simulink model "CICdatapowerfrompropagator_LoLaSat"  (R2022b)
settings: Solver=FixedStepAuto  StartTime=0.0  StopTime=t_sim  FixedStep=TimeStep  RelTol=1e-3
undefined symbols (not defined in the file or in its folder): date, eff_ADC1, eff_GPS, eff_OBC, eff_S, eff_UHF, EN_ADCS1, EN_GPS, EN_heat, EN_OBC, EN_S, EN_Thr, EN_UHF, juliandate, km, MODE, orbit, P_ADC, P_GPS, P_OBC, s
libraries: dspmathops x15, vrlib x8, aerolibutil x8, sharedtransform x7, simulink x4, sharedutil x4, simulink_extras x2, aerolibcelestial x1
settings Model: Creator=colpari  LastModifiedBy=lricc
settings SolverCC: AlgebraicLoopSolver=TrustRegion
settings DebuggingCC: UnconnectedInputMsg=warning  UnconnectedOutputMsg=warning  UnconnectedLineMsg=warning  SFMachineParentedDataDiag=warning
settings ModelReferenceCC: EnableRefExpFcnMdlSchedulingChecks=on
settings RTWCC: DLArmComputeVersion=19.05

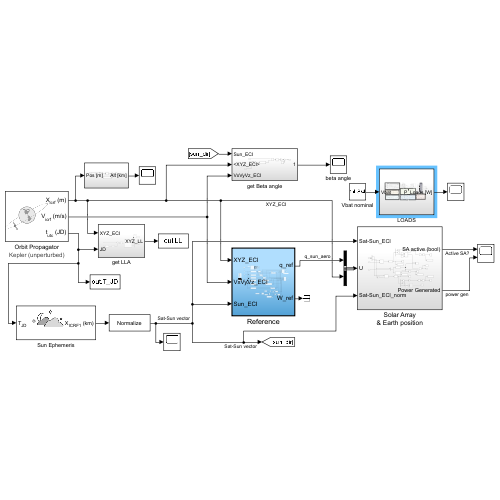
[thumbnail: Simulink's stored preview of the top-level diagram]
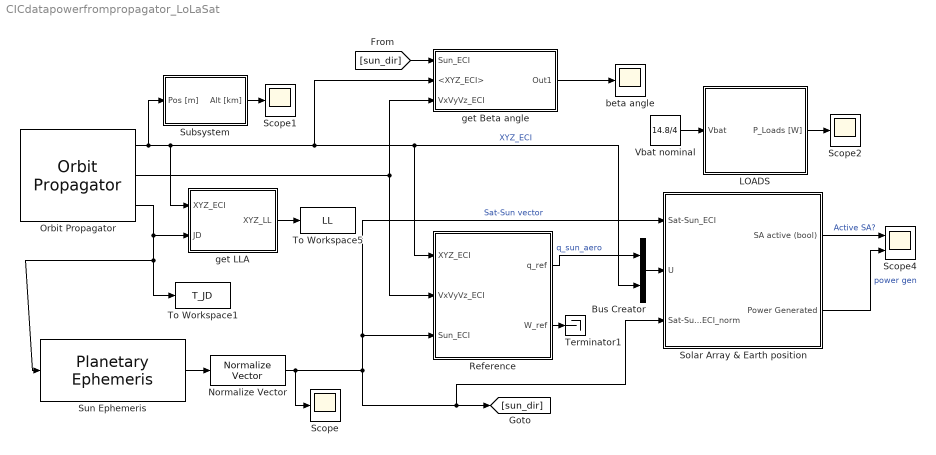
== system CICdatapowerfrompropagator_LoLaSat ==
  Bus Creator : BusCreator  Inputs=2
  LOADS : Subsystem
  Normalize Vector : vrlib/Utilities/Normalize Vector  maxzero=0
  Orbit Propagator : OrbitPropagator  startDate=juliandate(date.year, date.month, date.day, date.hour, date.minutes, date.seconds)  semiMajorAxis=orbit.a  eccentricity=orbit.e  inclination=orbit.i  raan=orbit.O  argPeriapsis=orbit.o  trueAnomaly=orbit.nu  inertialPosition=[3649700.0 3308200.0 -4676600.0]  inertialVelocity=[-2750.8 6666.4 2573.4]  fixedPosition=[-4142689.0 -2676864.7 -4669861.6]  fixedVelocity=[1452.7 -6720.7 2568.1]  customR=3396200  customMu=4.305e13  customJ2=1.0826269e-03  customOmega=4.06125949e-3
      settings: AttributesFormatString=%<propagator>
  Reference : Subsystem  TreatAsAtomicUnit=on
  Scope : Scope
  Scope1 : Scope
  Scope2 : Scope
  Scope4 : Scope  NumInputPorts=2
  Solar Array & Earth position : Subsystem
  Subsystem : Subsystem
  Sun Ephemeris : aerolibcelestial/Planetary Ephemeris  kmflag=km,km/s  epochflag=Julian date  de=DE405  nCenter=Earth  nTarget=Sun  errorflag=Error  velflag=off
  Terminator1 : Terminator
  To Workspace1 : ToWorkspace  VariableName=T_JD  SaveFormat=Timeseries  SampleTime=-1
  To Workspace5 : ToWorkspace  VariableName=LL  SaveFormat=Timeseries  SampleTime=-1
  Vbat nominal : Constant  Value=14.8/4
  beta angle : Scope
  get Beta angle : Subsystem
  get LLA : Subsystem
  wires:
  Reference/1(q_ref) -> Bus Creator/1  "q_sun_aero"
  Solar Array & Earth position/2(Power Generated) -> Scope4/2  "power gen"
  Orbit Propagator/2 -> Reference/2(VxVyVz_ECI), get Beta angle/3(VxVyVz_ECI)
  Normalize Vector/1 -> Scope/1, [sun_dir], Solar Array & Earth position/3(Sat-Sun_ECI_norm), Solar Array & Earth position/1(Sat-Sun_ECI), Reference/3(Sun_ECI)  "Sat-Sun vector"
  Bus Creator/1 -> Solar Array & Earth position/2(U)
  Solar Array & Earth position/1(SA active (bool)) -> Scope4/1  "Active SA?"
  Orbit Propagator/1 -> Subsystem/1(Pos [m]), get LLA/1(XYZ_ECI), Bus Creator/2, Reference/1(XYZ_ECI), get Beta angle/2(<XYZ_ECI>)  "XYZ_ECI"
  Orbit Propagator/3 -> To Workspace1/1, Sun Ephemeris/1, get LLA/2(JD)
  Reference/2(W_ref) -> Terminator1/1
  Sun Ephemeris/1 -> Normalize Vector/1
  get Beta angle/1(Out1) -> beta angle/1
  [sun_dir] -> get Beta angle/1(Sun_ECI)
  Subsystem/1(Alt [km]) -> Scope1/1
  get LLA/1(XYZ_LL) -> To Workspace5/1
  LOADS/1(P_Loads [W]) -> Scope2/1
  Vbat nominal/1 -> LOADS/1(Vbat)

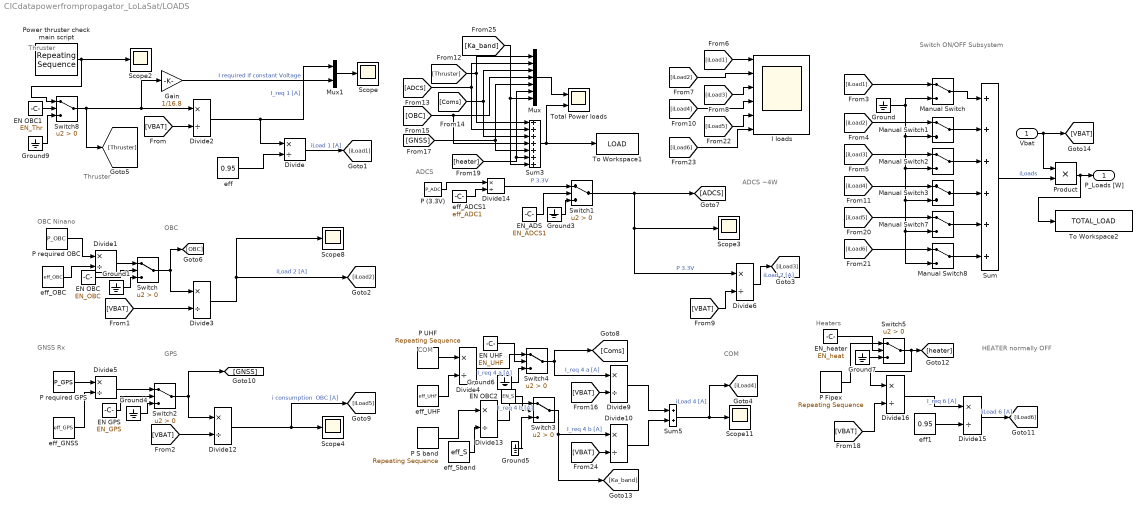
== system CICdatapowerfrompropagator_LoLaSat/LOADS ==
  note: Switch
      | ON/OFF
      | Subsystem
  note: Heaters
  note: COM
  note: ADCS
  note: OBC Ninano
  note: Thruster
  note: ADCS ~4W
  note: COM
  note: Thruster
  note: GNSS Rx
  note: GPS
  note: HEATER
      | normally
      | OFF
  note: OBC
  Vbat : Inport
  Divide{,1..6,9..10,12..16} (14 alike) : Product  Inputs=*/
  EN GPS : Constant  Value=EN_GPS
  EN OBC : Constant  Value=EN_OBC
  EN OBC1 : Constant  Value=EN_Thr
  EN OBC2 : Constant  Value=EN_S
  EN UHF : Constant  Value=EN_UHF
  EN_ADS : Constant  Value=EN_ADCS1
  EN_heater : Constant  Value=EN_heat
  Gain : Gain  Gain=1/16.8
  Ground{,1,3..7,9} (8 alike) : Ground
  I loads : Scope  NumInputPorts=6
  Manual Switch{,1..3,7..8} (6 alike) : ManualSwitch
  Mux : Mux  Inputs=7
  Mux1 : Mux  Inputs=2
  P (3.3V) : Constant  Value=P_ADC
  P Fipex : simulink/Sources/Repeating Sequence  rep_seq_t=t_Fi  rep_seq_y=p_Fi
  "P S band " : simulink/Sources/Repeating Sequence  rep_seq_t=t_tx_S  rep_seq_y=p_tx_S
  "P UHF " : simulink/Sources/Repeating Sequence  rep_seq_t=t_tx_UHF  rep_seq_y=p_tx_UHF
  P required GPS : Constant  Value=P_GPS
  P required OBC : Constant  Value=P_OBC
  Power thruster check main script : simulink/Sources/Repeating Sequence  rep_seq_t=t_thr  rep_seq_y=p_thr
  Product : Product
  Scope{,2..4,8,11} (6 alike) : Scope
  Sum : Sum  Inputs=++++++
  Sum3 : Sum  Inputs=+++++++
  Sum5 : Sum
  Switch{,1..5,8} (7 alike) : Switch  Criteria=u2 > Threshold  SaturateOnIntegerOverflow=off  InputSameDT=off
  To Workspace1 : ToWorkspace  VariableName=LOAD  SaveFormat=Timeseries  SampleTime=-1
  To Workspace2 : ToWorkspace  VariableName=TOTAL_LOAD  SaveFormat=Timeseries  SampleTime=-1
  Total Power loads : Scope  NumInputPorts=2
  eff : Constant  Value=0.95
  eff1 : Constant  Value=0.95
  "eff_ADCS1 " : Constant  Value=eff_ADC1
  eff_GNSS : Constant  Value=eff_GPS
  eff_OBC : Constant  Value=eff_OBC
  eff_Sband : Constant  Value=eff_S
  eff_UHF : Constant  Value=eff_UHF
  P_Loads [W] : Outport
  wires:
  Divide9/1 -> Sum5/1
  Sum5/1 -> [iLoad4], Scope11/1  "iLoad 4 [A]"
  Divide3/1 -> Scope8/1, [iLoad2]  "iLoad 2 [A]"
  Divide14/1 -> Switch1/1  "P 3.3V"
  Ground7/1 -> Switch5/3
  Power thruster check main script/1 -> Scope2/1, Switch8/1
  Sum3/1 -> Total Power loads/2, To Workspace1/1
  [Ka_band] -> Sum3/7, Mux/7
  Mux/1 -> Total Power loads/1
  EN OBC1/1 -> Switch8/2
  Divide4/1 -> Switch4/1  "I_req 4 a [A]"
  Ground5/1 -> Switch3/3
  EN_heater/1 -> Switch5/2
  EN_ADS/1 -> Switch1/2
  Divide10/1 -> Sum5/2
  Ground6/1 -> Switch4/3
  Divide13/1 -> Switch3/1  "I_req 4 b [A]"
  eff_UHF/1 -> Divide4/2
  Divide5/1 -> Switch2/1
  EN UHF/1 -> Switch4/2
  Divide15/1 -> [iLoad6]  "iLoad 6 [A]"
  Divide6/1 -> [iLoad3]  "iLoad 2 [A]"
  EN GPS/1 -> Switch2/2
  EN OBC2/1 -> Switch3/2
  Ground3/1 -> Switch1/3
  [Thruster] -> Sum3/1, Mux/1
  [iLoad6] -> I loads/6
  Manual Switch7/1 -> Sum/5
  Manual Switch8/1 -> Sum/6
  "P UHF "/1 -> Divide4/1
  Divide1/1 -> Switch/1
  eff/1 -> Divide/2
  [VBAT] -> Divide6/2
  Ground4/1 -> Switch2/3
  eff_Sband/1 -> Divide13/2
  [VBAT] -> Divide12/2
  Switch1/1 -> [ADCS], Divide6/1, Scope3/1  "P 3.3V"
  "eff_ADCS1 "/1 -> Divide14/2
  "P S band "/1 -> Divide13/1
  Ground1/1 -> Switch/3
  Switch2/1 -> [GNSS], Divide12/1
  P required OBC/1 -> Divide1/1
  Switch/1 -> Divide3/1, [OBC]
  Switch4/1 -> [Coms], Divide9/1  "I_req 4 a [A]"
  P required GPS/1 -> Divide5/1
  [iLoad3] -> I loads/3
  [iLoad5] -> I loads/5
  [VBAT] -> Divide9/2
  [iLoad6] -> Manual Switch8/1
  P Fipex/1 -> Switch5/1
  Switch8/1 -> [Thruster], Gain/1, Divide2/1
  [GNSS] -> Sum3/5, Mux/5
  [iLoad2] -> I loads/2
  [iLoad5] -> Manual Switch7/1
  Gain/1 -> Mux1/2  "I required if constant Voltage"
  eff_GNSS/1 -> Divide5/2
  [heater] -> Mux/6, Sum3/6
  [VBAT] -> Divide16/2
  Divide16/1 -> Divide15/1  "I_req 6 [A]"
  Divide12/1 -> [iLoad5], Scope4/1  "i consumption  OBC [A]"
  Manual Switch3/1 -> Sum/4
  [iLoad3] -> Manual Switch2/1
  [Coms] -> Sum3/3, Mux/3
  [iLoad4] -> I loads/4
  EN OBC/1 -> Switch/2
  [iLoad2] -> Manual Switch1/1
  [OBC] -> Sum3/4, Mux/4
  eff1/1 -> Divide15/2
  Manual Switch2/1 -> Sum/3
  Switch3/1 -> [Ka_band], Divide10/1  "I_req 4 b [A]"
  Manual Switch/1 -> Sum/1
  [ADCS] -> Sum3/2, Mux/2
  [VBAT] -> Divide10/2
  [iLoad4] -> Manual Switch3/1
  Mux1/1 -> Scope/1
  [iLoad1] -> Manual Switch/1
  Ground/1 -> Manual Switch/2, Manual Switch8/2, Manual Switch7/2, Manual Switch3/2, Manual Switch2/2, Manual Switch1/2
  Switch5/1 -> Divide16/1, [heater]
  Ground9/1 -> Switch8/3
  Divide2/1 -> Divide/1, Mux1/1  "I_req 1 [A]"
  [iLoad1] -> I loads/1
  [VBAT] -> Divide3/2
  Divide/1 -> [iLoad1]  "iLoad 1 [A]"
  eff_OBC/1 -> Divide1/2
  Manual Switch1/1 -> Sum/2
  [VBAT] -> Divide2/2
  P (3.3V)/1 -> Divide14/1
  Product/1 -> To Workspace2/1, P_Loads [W]/1
  Sum/1 -> Product/2  "iLoads"
  Vbat/1 -> Product/1, [VBAT]

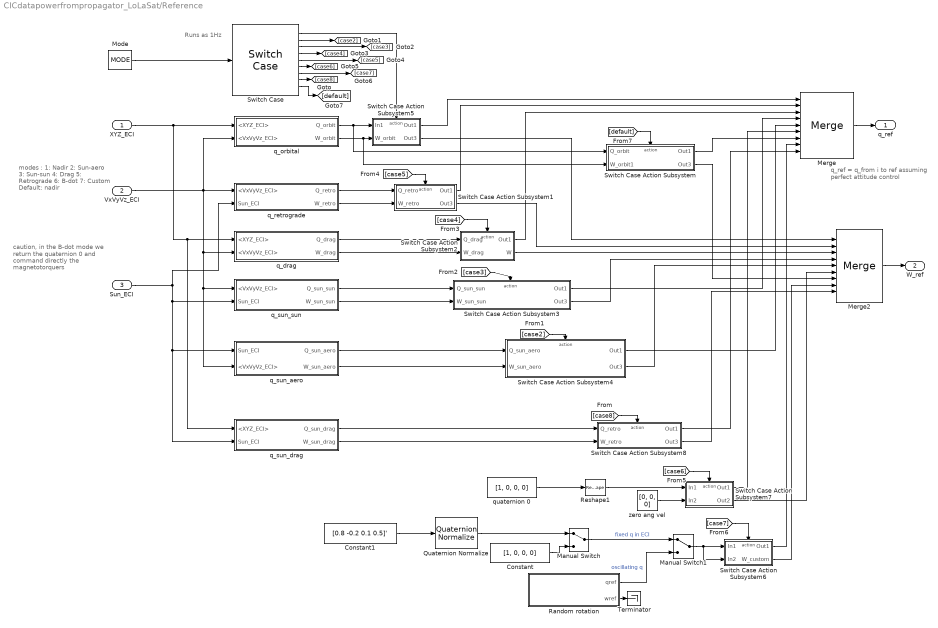
== system CICdatapowerfrompropagator_LoLaSat/Reference ==
  note: caution, in the B-dot mode we return the quaternion 0 and command directly the magnetotorquers
  note: modes :
      | 1: Nadir
      | 2: Sun-aero
      | 3: Sun-sun
      | 4: Drag
      | 5: Retrograde
      | 6: B-dot
      | 7: Custom
      | Default: nadir
  note: Runs as 1Hz
  note: q_ref  = q_from i to ref
      | assuming perfect attitude control
  XYZ_ECI : Inport
  VxVyVz_ECI : Inport  Port=2
  Sun_ECI : Inport  Port=3
  Constant : Constant  Value=[1, 0, 0, 0]
  Constant1 : Constant  Value=[0.8 -0.2 0.1 0.5]'
  Manual Switch : ManualSwitch
  Manual Switch1 : ManualSwitch
  Merge : Merge  Inputs=9
  Merge2 : Merge  Inputs=9
  Mode : Constant  Value=MODE  OutDataTypeStr=int8
  Quaternion Normalize : sharedutil/Quaternion Normalize  aMode=aMode
  Random rotation : Subsystem
  Reshape1 : Reshape  OutputDimensionality=Column vector (2-D)
  Switch Case : SwitchCase  CaseConditions={1, 2, 3, 4, 5, 6, 7, 8}
  Switch Case Action Subsystem : Subsystem  TreatAsAtomicUnit=on
  Switch Case Action Subsystem1 : Subsystem  TreatAsAtomicUnit=on
  Switch Case Action Subsystem2 : Subsystem  TreatAsAtomicUnit=on
  Switch Case Action Subsystem3 : Subsystem  TreatAsAtomicUnit=on
  Switch Case Action Subsystem4 : Subsystem  TreatAsAtomicUnit=on
  Switch Case Action Subsystem5 : Subsystem  TreatAsAtomicUnit=on
  Switch Case Action Subsystem6 : Subsystem  TreatAsAtomicUnit=on
  Switch Case Action Subsystem7 : Subsystem  TreatAsAtomicUnit=on
  Switch Case Action Subsystem8 : Subsystem  TreatAsAtomicUnit=on
  Terminator : Terminator
  q_drag : Subsystem
  q_orbital : Subsystem
  q_retrograde : Subsystem
  q_sun_aero : Subsystem
  q_sun_drag : Subsystem
  q_sun_sun : Subsystem
  quaternion 0 : Constant  Value=[1, 0, 0, 0]
  zero ang vel : Constant  Value=[0, 0, 0]
  q_ref : Outport  VectorParamsAs1DForOutWhenUnconnected=off
  W_ref : Outport  Port=2
  wires:
  q_sun_sun/1(Q_sun_sun) -> Switch Case Action Subsystem3/1(Q_sun_sun)
  Sun_ECI/1 -> q_retrograde/2(Sun_ECI), q_sun_drag/2(Sun_ECI), q_sun_aero/1(Sun_ECI), q_sun_sun/2(Sun_ECI)
  Mode/1 -> Switch Case/1
  q_sun_aero/1(Q_sun_aero) -> Switch Case Action Subsystem4/1(Q_sun_aero)
  Merge/1 -> q_ref/1
  quaternion 0/1 -> Reshape1/1
  VxVyVz_ECI/1 -> q_orbital/2(<VxVyVz_ECI>), q_retrograde/1(<VxVyVz_ECI>), q_drag/2(<VxVyVz_ECI>), q_sun_aero/2(<VxVyVz_ECI>), q_sun_sun/1(<VxVyVz_ECI>)
  q_orbital/1(Q_orbit) -> Switch Case Action Subsystem/1(Q_orbit), Switch Case Action Subsystem5/1(In1)
  q_retrograde/1(Q_retro) -> Switch Case Action Subsystem1/1(Q_retro)
  Reshape1/1 -> Switch Case Action Subsystem7/1(In1)
  Switch Case Action Subsystem5/1(Out1) -> Merge/1
  Switch Case Action Subsystem1/1(Out1) -> Merge/2
  Switch Case Action Subsystem2/1(Out1) -> Merge/3
  Switch Case Action Subsystem3/1(Out1) -> Merge/4
  Switch Case Action Subsystem4/1(Out1) -> Merge/5
  Switch Case Action Subsystem/1(Out1) -> Merge/7
  Switch Case Action Subsystem7/1(Out1) -> Merge/6
  Switch Case/1 -> Switch Case Action Subsystem5/Action
  Constant/1 -> Manual Switch/2
  Switch Case Action Subsystem6/1(Out1) -> Merge/8
  Constant1/1 -> Quaternion Normalize/1
  Quaternion Normalize/1 -> Manual Switch/1
  q_orbital/2(W_orbit) -> Switch Case Action Subsystem/2(W_orbit1), Switch Case Action Subsystem5/2(W_orbit)
  q_retrograde/2(W_retro) -> Switch Case Action Subsystem1/2(W_retro)
  q_sun_aero/2(W_sun_aero) -> Switch Case Action Subsystem4/2(W_sun_aero)
  q_sun_sun/2(W_sun_sun) -> Switch Case Action Subsystem3/2(W_sun_sun)
  Merge2/1 -> W_ref/1
  Switch Case Action Subsystem5/2(Out3) -> Merge2/1
  Switch Case Action Subsystem4/2(Out3) -> Merge2/5
  Switch Case Action Subsystem3/2(Out3) -> Merge2/4
  Switch Case Action Subsystem2/2(W) -> Merge2/3
  Switch Case Action Subsystem1/2(Out3) -> Merge2/2
  zero ang vel/1 -> Switch Case Action Subsystem7/2(In2)
  Switch Case Action Subsystem7/2(Out2) -> Merge2/6
  Switch Case Action Subsystem/2(Out3) -> Merge2/7
  Switch Case Action Subsystem6/2(W_custom) -> Merge2/8
  q_drag/1(Q_drag) -> Switch Case Action Subsystem2/1(Q_drag)
  q_drag/2(W_drag) -> Switch Case Action Subsystem2/2(W_drag)
  Manual Switch/1 -> Manual Switch1/1  "fixed q in ECI"
  Random rotation/1(qref) -> Manual Switch1/2  "oscillating q"
  Manual Switch1/1 -> Switch Case Action Subsystem6/2(In2), Switch Case Action Subsystem6/1(In1)
  Random rotation/2(wref) -> Terminator/1
  XYZ_ECI/1 -> q_sun_drag/1(<XYZ_ECI>), q_drag/1(<XYZ_ECI>), q_orbital/1(<XYZ_ECI>)
  q_sun_drag/1(Q_sun_drag) -> Switch Case Action Subsystem8/1(Q_retro)
  q_sun_drag/2(W_sun_drag) -> Switch Case Action Subsystem8/2(W_retro)
  Switch Case/8 -> [case8]
  [case8] -> Switch Case Action Subsystem8/Action
  Switch Case Action Subsystem8/1(Out1) -> Merge/9
  Switch Case Action Subsystem8/2(Out3) -> Merge2/9
  Switch Case/2 -> [case2]
  [case2] -> Switch Case Action Subsystem4/Action
  Switch Case/3 -> [case3]
  [case3] -> Switch Case Action Subsystem3/Action
  Switch Case/4 -> [case4]
  [case4] -> Switch Case Action Subsystem2/Action
  Switch Case/5 -> [case5]
  [case5] -> Switch Case Action Subsystem1/Action
  Switch Case/6 -> [case6]
  [case6] -> Switch Case Action Subsystem7/Action
  Switch Case/7 -> [case7]
  [case7] -> Switch Case Action Subsystem6/Action
  Switch Case/9 -> [default]
  [default] -> Switch Case Action Subsystem/Action

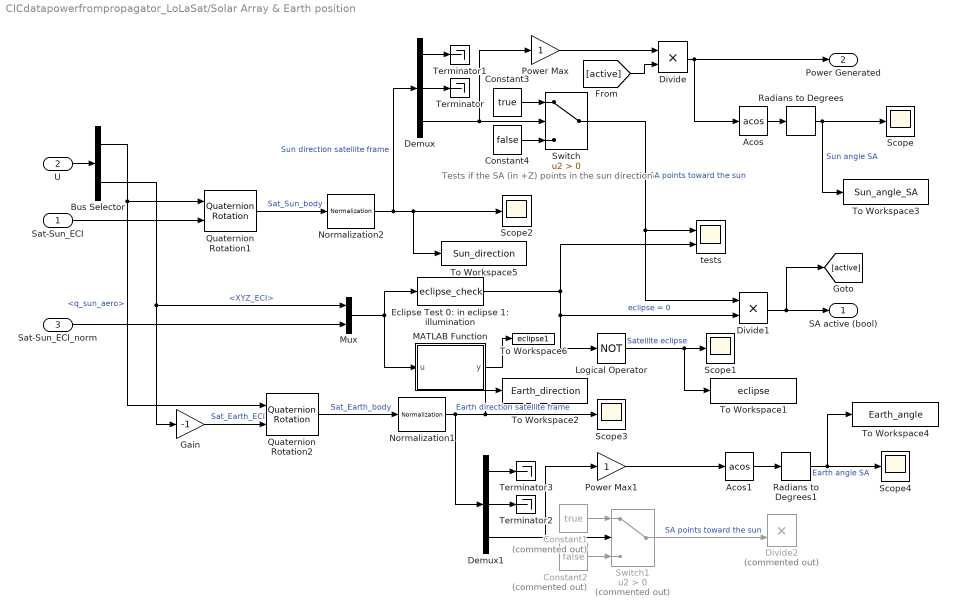
== system CICdatapowerfrompropagator_LoLaSat/Solar Array & Earth position ==
  note: Tests if the SA (in +Z) points in the sun direction
  Sat-Sun_ECI : Inport
  U : Inport  Port=2
  Sat-Sun_ECI_norm : Inport  Port=3
  Acos : Trigonometry  Operator=acos
  Acos1 : Trigonometry  Operator=acos
  Bus Selector : BusSelector  OutputSignals=q_sun_aero,XYZ_ECI
  Constant1 : Constant  Commented=on  Value=true
  Constant2 : Constant  Commented=on  Value=false
  Constant3 : Constant  Value=true
  Constant4 : Constant  Value=false
  Demux : Demux  Outputs=3
  Demux1 : Demux  Outputs=3
  Divide : Product  Inputs=**
  Divide1 : Product  Inputs=**
  Divide2 : Product  Commented=on  Inputs=**
  Eclipse Test 0: in eclipse 1: illumination : MATLABFcn  MATLABFcn=eclipse_check
  Gain : Gain  Gain=-1
  Logical Operator : Logic  Operator=NOT  AllPortsSameDT=off
  MATLAB Function : MATLAB Function  TreatAsAtomicUnit=on
  Mux : Mux  Inputs=2
  Normalization1 : dspmathops/Normalization  NormType=2-norm  Bias=1e-10  NormOver=Each column  Dimension=1  roundingMode=Floor  overflowMode=off  accumDataTypeStr=Inherit: Same as product output  accumLastDataTypeStr=Inherit: Same as product output  outputDataTypeStr=Inherit: Same as product output  outputMin=[]  outputMax=[]  outputLastDataTypeStr=Inherit: Same as product output
  Normalization2 : dspmathops/Normalization  NormType=2-norm  Bias=1e-10  NormOver=Each column  Dimension=1  roundingMode=Floor  overflowMode=off  accumDataTypeStr=Inherit: Same as product output  accumLastDataTypeStr=Inherit: Same as product output  outputDataTypeStr=Inherit: Same as product output  outputMin=[]  outputMax=[]  outputLastDataTypeStr=Inherit: Same as product output
  Power Max : Gain
  Power Max1 : Gain
  Quaternion Rotation1 : aerolibutil/Quaternion Rotation
  Quaternion Rotation2 : aerolibutil/Quaternion Rotation
  Radians to Degrees : simulink_extras/Transformations/Radians to Degrees
  Radians to Degrees1 : simulink_extras/Transformations/Radians to Degrees
  Scope{,1..4} (5 alike) : Scope
  Switch : Switch  Criteria=u2 > Threshold  SaturateOnIntegerOverflow=off  InputSameDT=off
  Switch1 : Switch  Commented=on  Criteria=u2 > Threshold  SaturateOnIntegerOverflow=off  InputSameDT=off
  Terminator{,1..3} (4 alike) : Terminator
  To Workspace1 : ToWorkspace  VariableName=eclipse  SaveFormat=Timeseries  SampleTime=-1
  To Workspace2 : ToWorkspace  VariableName=Earth_direction  SaveFormat=Timeseries  SampleTime=-1
  To Workspace3 : ToWorkspace  VariableName=Sun_angle_SA  SaveFormat=Timeseries  SampleTime=-1
  To Workspace4 : ToWorkspace  VariableName=Earth_angle  SaveFormat=Timeseries  SampleTime=-1
  To Workspace5 : ToWorkspace  VariableName=Sun_direction  SaveFormat=Timeseries  SampleTime=-1
  To Workspace6 : ToWorkspace  VariableName=eclipse1  SaveFormat=Timeseries  SampleTime=-1
  tests : Scope  NumInputPorts=2
  SA active (bool) : Outport  VectorParamsAs1DForOutWhenUnconnected=off
  Power Generated : Outport  Port=2
  wires:
  Switch/1 -> Divide1/1, tests/1  "SA points toward the sun"
  U/1 -> Bus Selector/1
  Sat-Sun_ECI/1 -> Quaternion Rotation1/2
  Bus Selector/1 -> Quaternion Rotation2/1, Quaternion Rotation1/1  "<q_sun_aero>"
  Quaternion Rotation1/1 -> Normalization2/1  "Sat_Sun_body"
  Demux/3 -> Power Max/1, Switch/2
  Constant3/1 -> Switch/1
  Demux/2 -> Terminator/1
  Demux/1 -> Terminator1/1
  Bus Selector/2 -> Gain/1, Mux/1  "<XYZ_ECI>"
  Divide1/1 -> [active], SA active (bool)/1
  Constant4/1 -> Switch/3
  Normalization2/1 -> To Workspace5/1, Scope2/1, Demux/1  "Sun direction satellite frame"
  Divide/1 -> Acos/1, Power Generated/1
  Power Max/1 -> Divide/1
  [active] -> Divide/2
  Sat-Sun_ECI_norm/1 -> Mux/2
  Mux/1 -> Eclipse Test 0: in eclipse 1: illumination/1, MATLAB Function/1(u)
  Eclipse Test 0: in eclipse 1: illumination/1 -> Logical Operator/1, Divide1/2, tests/2  "eclipse = 0"
  Acos/1 -> Radians to Degrees/1
  Radians to Degrees/1 -> To Workspace3/1, Scope/1  "Sun angle SA"
  Logical Operator/1 -> To Workspace1/1, Scope1/1  "Satellite eclipse"
  Gain/1 -> Quaternion Rotation2/2  "Sat_Earth_ECI"
  Quaternion Rotation2/1 -> Normalization1/1  "Sat_Earth_body"
  Power Max1/1 -> Acos1/1
  Demux1/3 -> Power Max1/1, Switch1/2
  Demux1/2 -> Terminator2/1
  Normalization1/1 -> Demux1/1, To Workspace2/1, Scope3/1  "Earth direction satellite frame"
  Constant2/1 -> Switch1/3
  Constant1/1 -> Switch1/1
  Switch1/1 -> Divide2/2  "SA points toward the sun"
  Demux1/1 -> Terminator3/1
  Acos1/1 -> Radians to Degrees1/1
  Radians to Degrees1/1 -> To Workspace4/1, Scope4/1  "Earth angle SA"
  MATLAB Function/1(y) -> To Workspace6/1

== system CICdatapowerfrompropagator_LoLaSat/Subsystem ==
  Pos [m] : Inport
  Constant : Constant  Value=orbit.R_earth
  Dot Product : DotProduct  OutDataTypeStr=Inherit: Inherit via internal rule
  Gain : Gain  Gain=1e-3
  Sqrt : Sqrt
  Sum : Sum  Inputs=|+-
  Alt [km] : Outport
  wires:
  Dot Product/1 -> Sqrt/1
  Pos [m]/1 -> Dot Product/2, Dot Product/1
  Sqrt/1 -> Sum/1
  Constant/1 -> Sum/2
  Sum/1 -> Gain/1
  Gain/1 -> Alt [km]/1

== system CICdatapowerfrompropagator_LoLaSat/get Beta angle ==
  Sun_ECI : Inport
  <XYZ_ECI> : Inport  Port=2
  VxVyVz_ECI : Inport  Port=3
  Acos : Trigonometry  Operator=acos
  Constant1 : Constant  Value=90
  Cross Product : vrlib/Utilities/Cross Product
  Dot Product : DotProduct  OutDataTypeStr=Inherit: Inherit via internal rule
  Gain : Gain  Gain=180/pi
  Normalize Vector2 : vrlib/Utilities/Normalize Vector  maxzero=0
  Sum : Sum  Inputs=|-+
  Out1 : Outport
  wires:
  Normalize Vector2/1 -> Dot Product/2  "x"
  Constant1/1 -> Sum/2
  Cross Product/1 -> Normalize Vector2/1
  Sun_ECI/1 -> Dot Product/1
  Dot Product/1 -> Acos/1
  Acos/1 -> Gain/1
  Gain/1 -> Sum/1
  Sum/1 -> Out1/1
  <XYZ_ECI>/1 -> Cross Product/1
  VxVyVz_ECI/1 -> Cross Product/2

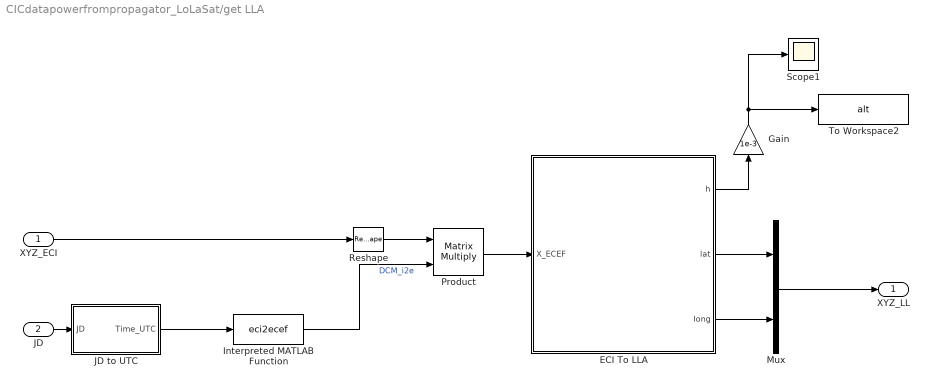
== system CICdatapowerfrompropagator_LoLaSat/get LLA ==
  XYZ_ECI : Inport
  JD : Inport  Port=2
  ECI To LLA : MATLAB Function  TreatAsAtomicUnit=on
  Gain : Gain  Gain=1e-3
  Interpreted MATLAB Function : MATLABFcn  MATLABFcn=eci2ecef  OutputDimensions=[3,3]  Output1D=off
  JD to UTC : MATLAB Function  TreatAsAtomicUnit=on
  Mux : Mux  Inputs=2
  Product : Product  Multiplication=Matrix(*)
  Reshape : Reshape  OutputDimensionality=Row vector (2-D)
  Scope1 : Scope
  To Workspace2 : ToWorkspace  VariableName=alt  SaveFormat=Timeseries  SampleTime=-1
  XYZ_LL : Outport
  wires:
  JD to UTC/1(Time_UTC) -> Interpreted MATLAB Function/1
  JD/1 -> JD to UTC/1(JD)
  Product/1 -> ECI To LLA/1(X_ECEF)
  ECI To LLA/2(lat) -> Mux/1
  ECI To LLA/3(long) -> Mux/2
  ECI To LLA/1(h) -> Gain/1
  Reshape/1 -> Product/1
  XYZ_ECI/1 -> Reshape/1
  Interpreted MATLAB Function/1 -> Product/2  "DCM_i2e"
  Gain/1 -> Scope1/1, To Workspace2/1
  Mux/1 -> XYZ_LL/1

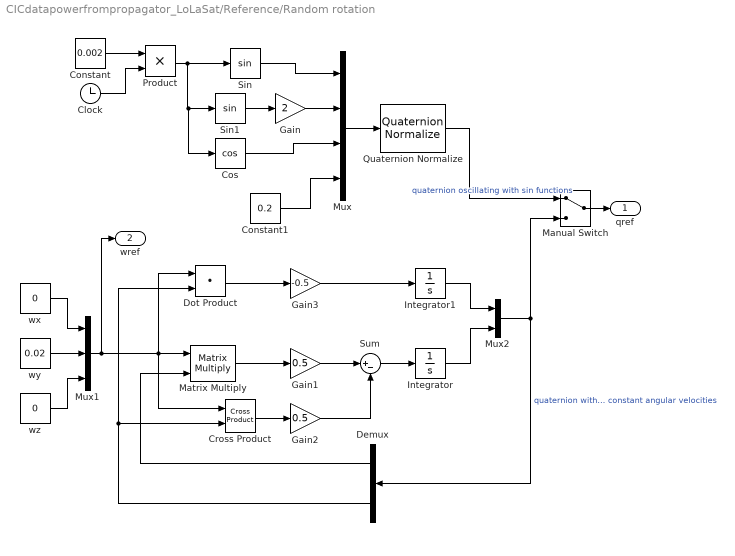
== system CICdatapowerfrompropagator_LoLaSat/Reference/Random rotation ==
  Clock : Clock
      settings: Decimation=TimeStep
  Constant : Constant  Value=0.002
  Constant1 : Constant  Value=0.2
  Cos : Trigonometry  Operator=cos
  Cross Product : vrlib/Utilities/Cross Product
  Demux : Demux  Outputs=[1;3]
  Dot Product : DotProduct  OutDataTypeStr=Inherit: Inherit via internal rule
  Gain : Gain  Gain=2
  Gain1 : Gain  Gain=0.5
  Gain2 : Gain  Gain=0.5
  Gain3 : Gain  Gain=-0.5
  Integrator : Integrator  InitialCondition=[0;0;0]
  Integrator1 : Integrator  InitialCondition=1
  Manual Switch : ManualSwitch
  Matrix Multiply : Product  Multiplication=Matrix(*)
  Mux : Mux
  Mux1 : Mux  Inputs=3
  Mux2 : Mux  Inputs=[1;3]
  Product : Product
  Quaternion Normalize : sharedutil/Quaternion Normalize  aMode=aMode
  Sin : Trigonometry
  Sin1 : Trigonometry
  Sum : Sum  Inputs=|+-
  wx : Constant  Value=0
  wy : Constant  Value=0.02
  wz : Constant  Value=0
  qref : Outport
  wref : Outport  Port=2
  wires:
  Mux/1 -> Quaternion Normalize/1
  Quaternion Normalize/1 -> Manual Switch/1  "quaternion oscillating with sin functions"
  Constant/1 -> Product/1
  Clock/1 -> Product/2
  Product/1 -> Cos/1, Sin1/1, Sin/1
  Sin/1 -> Mux/1
  Sin1/1 -> Gain/1
  Gain/1 -> Mux/2
  Cos/1 -> Mux/3
  Constant1/1 -> Mux/4
  Manual Switch/1 -> qref/1
  wx/1 -> Mux1/1
  wy/1 -> Mux1/2
  wz/1 -> Mux1/3
  Mux1/1 -> wref/1, Dot Product/1, Cross Product/1, Matrix Multiply/1
  Matrix Multiply/1 -> Gain1/1
  Gain1/1 -> Sum/1
  Sum/1 -> Integrator/1
  Integrator/1 -> Mux2/2
  Mux2/1 -> Demux/1, Manual Switch/2  "quaternion with constant angular velocities"
  Demux/1 -> Matrix Multiply/2
  Cross Product/1 -> Gain2/1
  Gain2/1 -> Sum/2
  Dot Product/1 -> Gain3/1
  Gain3/1 -> Integrator1/1
  Integrator1/1 -> Mux2/1
  Demux/2 -> Cross Product/2, Dot Product/2

== system CICdatapowerfrompropagator_LoLaSat/Reference/Switch Case Action Subsystem ==
  Q_orbit : Inport
  W_orbit1 : Inport  Port=2
  Action Port : ActionPort  ActionPortLabel=default:
  Out1 : Outport  VectorParamsAs1DForOutWhenUnconnected=off
  Out3 : Outport  Port=2  VectorParamsAs1DForOutWhenUnconnected=off
  wires:
  Q_orbit/1 -> Out1/1
  W_orbit1/1 -> Out3/1

== system CICdatapowerfrompropagator_LoLaSat/Reference/Switch Case Action Subsystem1 ==
  Q_retro : Inport
  W_retro : Inport  Port=2
  Action Port : ActionPort  ActionPortLabel=case [ 5 ]:
  Out1 : Outport  VectorParamsAs1DForOutWhenUnconnected=off
  Out3 : Outport  Port=2  VectorParamsAs1DForOutWhenUnconnected=off
  wires:
  Q_retro/1 -> Out1/1
  W_retro/1 -> Out3/1

== system CICdatapowerfrompropagator_LoLaSat/Reference/Switch Case Action Subsystem2 ==
  note: q from I to O + rotation
  Q_drag : Inport
  W_drag : Inport  Port=2
  Action Port : ActionPort  ActionPortLabel=case [ 4 ]:
  Out1 : Outport  VectorParamsAs1DForOutWhenUnconnected=off
  W : Outport  Port=2
  wires:
  Q_drag/1 -> Out1/1
  W_drag/1 -> W/1

== system CICdatapowerfrompropagator_LoLaSat/Reference/Switch Case Action Subsystem3 ==
  Q_sun_sun : Inport
  W_sun_sun : Inport  Port=2
  Action Port : ActionPort  ActionPortLabel=case [ 3 ]:
  Out1 : Outport  VectorParamsAs1DForOutWhenUnconnected=off
  Out3 : Outport  Port=2  VectorParamsAs1DForOutWhenUnconnected=off
  wires:
  Q_sun_sun/1 -> Out1/1
  W_sun_sun/1 -> Out3/1

== system CICdatapowerfrompropagator_LoLaSat/Reference/Switch Case Action Subsystem4 ==
  Q_sun_aero : Inport
  W_sun_aero : Inport  Port=2
  Action Port : ActionPort  ActionPortLabel=case [ 2 ]:
  Out1 : Outport  VectorParamsAs1DForOutWhenUnconnected=off
  Out3 : Outport  Port=2  VectorParamsAs1DForOutWhenUnconnected=off
  wires:
  Q_sun_aero/1 -> Out1/1
  W_sun_aero/1 -> Out3/1

== system CICdatapowerfrompropagator_LoLaSat/Reference/Switch Case Action Subsystem5 ==
  In1 : Inport
  W_orbit : Inport  Port=2
  Action Port : ActionPort  ActionPortLabel=case [ 1 ]:
  Out1 : Outport  VectorParamsAs1DForOutWhenUnconnected=off
  Out3 : Outport  Port=2  VectorParamsAs1DForOutWhenUnconnected=off
  wires:
  In1/1 -> Out1/1
  W_orbit/1 -> Out3/1

== system CICdatapowerfrompropagator_LoLaSat/Reference/Switch Case Action Subsystem6 ==
  In1 : Inport
  In2 : Inport  Port=2
  Action Port : ActionPort  ActionPortLabel=case [ 7 ]:
  Derivative : Derivative
  Matrix Multiply : Product  Multiplication=Matrix(*)
  Quaternions to Direction Cosine Matrix : sharedtransform/Quaternions to  Direction Cosine Matrix  aMode=aMode
  Transpose : Math  Operator=transpose
  Transpose1 : Math  Operator=transpose
  gets vector from Skew Matrix : MATLABFcn  MATLABFcn=vec_from_skew
  Out1 : Outport  VectorParamsAs1DForOutWhenUnconnected=off
  W_custom : Outport  Port=2
  wires:
  In1/1 -> Out1/1
  In2/1 -> Quaternions to Direction Cosine Matrix/1
  Quaternions to Direction Cosine Matrix/1 -> Transpose1/1
  Matrix Multiply/1 -> gets vector from Skew Matrix/1
  Transpose/1 -> Derivative/1
  gets vector from Skew Matrix/1 -> W_custom/1
  Derivative/1 -> Matrix Multiply/1
  Transpose1/1 -> Transpose/1, Matrix Multiply/2

== system CICdatapowerfrompropagator_LoLaSat/Reference/Switch Case Action Subsystem7 ==
  In1 : Inport
  In2 : Inport  Port=2
  Action Port : ActionPort  ActionPortLabel=case [ 6 ]:
  Out1 : Outport  VectorParamsAs1DForOutWhenUnconnected=off
  Out2 : Outport  Port=2  VectorParamsAs1DForOutWhenUnconnected=off
  wires:
  In1/1 -> Out1/1
  In2/1 -> Out2/1

== system CICdatapowerfrompropagator_LoLaSat/Reference/Switch Case Action Subsystem8 ==
  Q_retro : Inport
  W_retro : Inport  Port=2
  Action Port : ActionPort  ActionPortLabel=case [ 8 ]:
  Out1 : Outport  VectorParamsAs1DForOutWhenUnconnected=off
  Out3 : Outport  Port=2  VectorParamsAs1DForOutWhenUnconnected=off
  wires:
  Q_retro/1 -> Out1/1
  W_retro/1 -> Out3/1

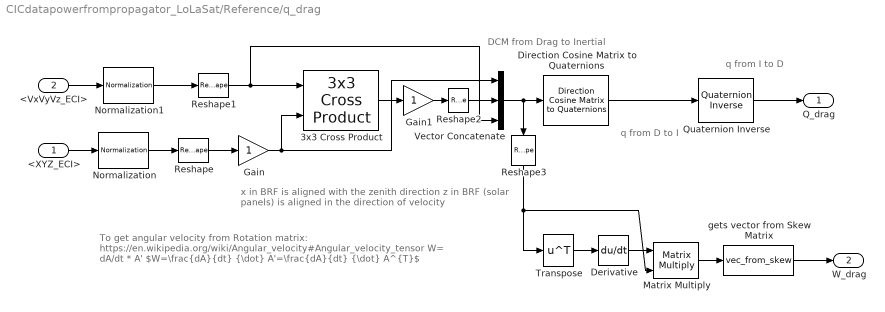
== system CICdatapowerfrompropagator_LoLaSat/Reference/q_drag ==
  note: x in BRF is aligned with the zenith direction
      | z in BRF (solar panels) is aligned in the direction of velocity
  note: DCM from Drag to Inertial
  note: q from D to I
  note: q from I to D
  note: To get angular velocity from Rotation matrix:
      | https://en.wikipedia.org/wiki/Angular_velocity#Angular_velocity_tensor
      | W= dA/dt * A'
      | $W=\frac{dA}{dt} {\dot} A'=\frac{dA}{dt} {\dot} A^{T}$
  <XYZ_ECI> : Inport
  <VxVyVz_ECI> : Inport  Port=2
  3x3 Cross Product : sharedutil/3x3 Cross Product  aMode=aMode
  Derivative : Derivative
  Direction Cosine Matrix to Quaternions : sharedtransform/Direction Cosine Matrix  to Quaternions  aMode=0  action=None  tolerance=eps(2)
  Gain : Gain
  Gain1 : Gain
  Matrix Multiply : Product  Multiplication=Matrix(*)
  Normalization : dspmathops/Normalization  NormType=2-norm  Bias=1e-10  NormOver=Each column  Dimension=1  roundingMode=Floor  overflowMode=off  accumDataTypeStr=Inherit: Same as product output  accumLastDataTypeStr=Inherit: Same as product output  outputDataTypeStr=Inherit: Same as product output  outputMin=[]  outputMax=[]  outputLastDataTypeStr=Inherit: Same as product output
  Normalization1 : dspmathops/Normalization  NormType=2-norm  Bias=1e-10  NormOver=Each column  Dimension=1  roundingMode=Floor  overflowMode=off  accumDataTypeStr=Inherit: Same as product output  accumLastDataTypeStr=Inherit: Same as product output  outputDataTypeStr=Inherit: Same as product output  outputMin=[]  outputMax=[]  outputLastDataTypeStr=Inherit: Same as product output
  Quaternion Inverse : aerolibutil/Quaternion Inverse
  Reshape : Reshape  OutputDimensionality=Column vector (2-D)
  Reshape1 : Reshape  OutputDimensionality=Column vector (2-D)
  Reshape2 : Reshape  OutputDimensionality=Column vector (2-D)
  Reshape3 : Reshape  OutputDimensionality=Customize  OutputDimensions=[3,3]
  Transpose : Math  Operator=transpose
  Vector Concatenate : Concatenate  NumInputs=3  Mode=Multidimensional array  ConcatenateDimension=2
  gets vector from Skew Matrix : MATLABFcn  MATLABFcn=vec_from_skew
  Q_drag : Outport  VectorParamsAs1DForOutWhenUnconnected=off
  W_drag : Outport  Port=2
  wires:
  Normalization/1 -> Reshape/1
  Normalization1/1 -> Reshape1/1
  <VxVyVz_ECI>/1 -> Normalization1/1
  Reshape1/1 -> Vector Concatenate/3, 3x3 Cross Product/1
  <XYZ_ECI>/1 -> Normalization/1
  Reshape/1 -> Gain/1
  Gain/1 -> Vector Concatenate/1, 3x3 Cross Product/2
  Direction Cosine Matrix to Quaternions/1 -> Quaternion Inverse/1
  3x3 Cross Product/1 -> Gain1/1
  Gain1/1 -> Reshape2/1
  Quaternion Inverse/1 -> Q_drag/1
  Vector Concatenate/1 -> Reshape3/1, Direction Cosine Matrix to Quaternions/1
  gets vector from Skew Matrix/1 -> W_drag/1
  Matrix Multiply/1 -> gets vector from Skew Matrix/1
  Transpose/1 -> Derivative/1
  Derivative/1 -> Matrix Multiply/1
  Reshape2/1 -> Vector Concatenate/2
  Reshape3/1 -> Matrix Multiply/2, Transpose/1

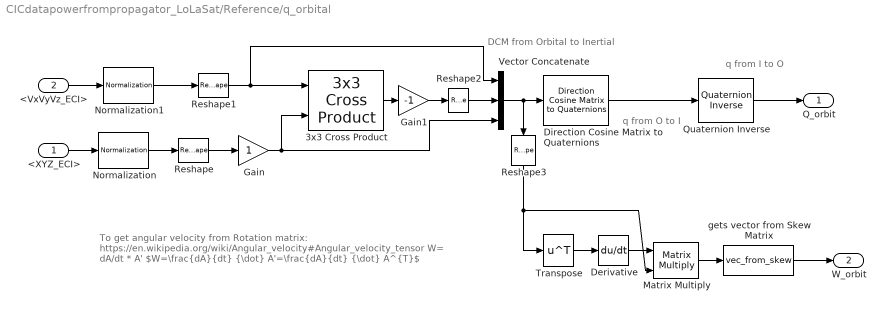
== system CICdatapowerfrompropagator_LoLaSat/Reference/q_orbital ==
  note: DCM from Orbital to Inertial
  note: q from O to I
  note: q from I to O
  note: To get angular velocity from Rotation matrix:
      | https://en.wikipedia.org/wiki/Angular_velocity#Angular_velocity_tensor
      | W= dA/dt * A'
      | $W=\frac{dA}{dt} {\dot} A'=\frac{dA}{dt} {\dot} A^{T}$
  <XYZ_ECI> : Inport
  <VxVyVz_ECI> : Inport  Port=2
  3x3 Cross Product : sharedutil/3x3 Cross Product  aMode=aMode
  Derivative : Derivative
  Direction Cosine Matrix to Quaternions : sharedtransform/Direction Cosine Matrix  to Quaternions  aMode=0  action=None  tolerance=eps(2)
  Gain : Gain
  Gain1 : Gain  Gain=-1
  Matrix Multiply : Product  Multiplication=Matrix(*)
  Normalization : dspmathops/Normalization  NormType=2-norm  Bias=1e-10  NormOver=Each column  Dimension=1  roundingMode=Floor  overflowMode=off  accumDataTypeStr=Inherit: Same as product output  accumLastDataTypeStr=Inherit: Same as product output  outputDataTypeStr=Inherit: Same as product output  outputMin=[]  outputMax=[]  outputLastDataTypeStr=Inherit: Same as product output
  Normalization1 : dspmathops/Normalization  NormType=2-norm  Bias=1e-10  NormOver=Each column  Dimension=1  roundingMode=Floor  overflowMode=off  accumDataTypeStr=Inherit: Same as product output  accumLastDataTypeStr=Inherit: Same as product output  outputDataTypeStr=Inherit: Same as product output  outputMin=[]  outputMax=[]  outputLastDataTypeStr=Inherit: Same as product output
  Quaternion Inverse : aerolibutil/Quaternion Inverse
  Reshape : Reshape  OutputDimensionality=Column vector (2-D)
  Reshape1 : Reshape  OutputDimensionality=Column vector (2-D)
  Reshape2 : Reshape  OutputDimensionality=Column vector (2-D)
  Reshape3 : Reshape  OutputDimensionality=Customize  OutputDimensions=[3,3]
  Transpose : Math  Operator=transpose
  Vector Concatenate : Concatenate  NumInputs=3  Mode=Multidimensional array  ConcatenateDimension=2
  gets vector from Skew Matrix : MATLABFcn  MATLABFcn=vec_from_skew
  Q_orbit : Outport  VectorParamsAs1DForOutWhenUnconnected=off
  W_orbit : Outport  Port=2
  wires:
  Normalization/1 -> Reshape/1
  Normalization1/1 -> Reshape1/1
  <VxVyVz_ECI>/1 -> Normalization1/1
  Reshape1/1 -> 3x3 Cross Product/1, Vector Concatenate/1
  <XYZ_ECI>/1 -> Normalization/1
  Reshape/1 -> Gain/1
  Gain/1 -> 3x3 Cross Product/2, Vector Concatenate/3
  Direction Cosine Matrix to Quaternions/1 -> Quaternion Inverse/1
  3x3 Cross Product/1 -> Gain1/1
  Gain1/1 -> Reshape2/1
  Quaternion Inverse/1 -> Q_orbit/1
  Vector Concatenate/1 -> Reshape3/1, Direction Cosine Matrix to Quaternions/1
  gets vector from Skew Matrix/1 -> W_orbit/1
  Matrix Multiply/1 -> gets vector from Skew Matrix/1
  Transpose/1 -> Derivative/1
  Derivative/1 -> Matrix Multiply/1
  Reshape2/1 -> Vector Concatenate/2
  Reshape3/1 -> Matrix Multiply/2, Transpose/1

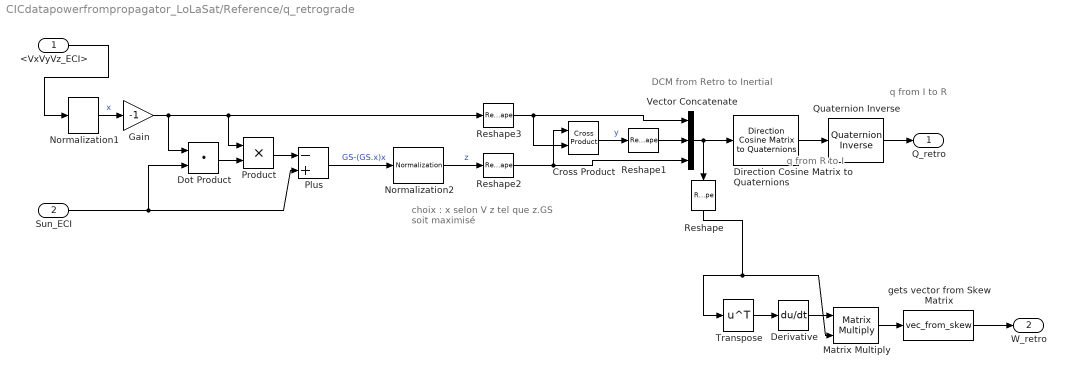
== system CICdatapowerfrompropagator_LoLaSat/Reference/q_retrograde ==
  note: q from I to R
  note: q from R to I
  note: DCM from Retro to Inertial
  note: choix :
      | x selon V
      | z tel que z.GS soit maximisé
  <VxVyVz_ECI> : Inport
  Sun_ECI : Inport  Port=2
  Cross Product : vrlib/Utilities/Cross Product
  Derivative : Derivative
  Direction Cosine Matrix to Quaternions : sharedtransform/Direction Cosine Matrix  to Quaternions  aMode=0  action=None  tolerance=eps(2)
  Dot Product : DotProduct  OutDataTypeStr=Inherit: Inherit via internal rule
  Gain : Gain  Gain=-1
  Matrix Multiply : Product  Multiplication=Matrix(*)
  Normalization1 : dspmathops/Normalization  NormType=2-norm  Bias=1e-10  NormOver=Each column  Dimension=1  roundingMode=Floor  overflowMode=off  accumDataTypeStr=Inherit: Same as product output  accumLastDataTypeStr=Inherit: Same as product output  outputDataTypeStr=Inherit: Same as product output  outputMin=[]  outputMax=[]  outputLastDataTypeStr=Inherit: Same as product output
  Normalization2 : dspmathops/Normalization  NormType=2-norm  Bias=1e-10  NormOver=Each column  Dimension=1  roundingMode=Floor  overflowMode=off  accumDataTypeStr=Inherit: Same as product output  accumLastDataTypeStr=Inherit: Same as product output  outputDataTypeStr=Inherit: Same as product output  outputMin=[]  outputMax=[]  outputLastDataTypeStr=Inherit: Same as product output
  Plus : Sum  Inputs=-+
  Product : Product
  Quaternion Inverse : aerolibutil/Quaternion Inverse
  Reshape : Reshape  OutputDimensionality=Customize  OutputDimensions=[3,3]
  Reshape1 : Reshape  OutputDimensionality=Column vector (2-D)
  Reshape2 : Reshape  OutputDimensionality=Column vector (2-D)
  Reshape3 : Reshape  OutputDimensionality=Column vector (2-D)
  Transpose : Math  Operator=transpose
  Vector Concatenate : Concatenate  NumInputs=3  Mode=Multidimensional array  ConcatenateDimension=2
  gets vector from Skew Matrix : MATLABFcn  MATLABFcn=vec_from_skew
  Q_retro : Outport  VectorParamsAs1DForOutWhenUnconnected=off
  W_retro : Outport  Port=2
  wires:
  Quaternion Inverse/1 -> Q_retro/1
  Reshape2/1 -> Vector Concatenate/3, Cross Product/1
  Reshape3/1 -> Vector Concatenate/1, Cross Product/2
  Product/1 -> Plus/1
  Dot Product/1 -> Product/2
  Cross Product/1 -> Reshape1/1  "y"
  Normalization2/1 -> Reshape2/1  "z"
  Plus/1 -> Normalization2/1  "GS-(GS.x)x"
  Sun_ECI/1 -> Dot Product/2, Plus/2
  Direction Cosine Matrix to Quaternions/1 -> Quaternion Inverse/1
  Normalization1/1 -> Gain/1  "x"
  <VxVyVz_ECI>/1 -> Normalization1/1
  Reshape1/1 -> Vector Concatenate/2
  Gain/1 -> Dot Product/1, Product/1, Reshape3/1
  Vector Concatenate/1 -> Direction Cosine Matrix to Quaternions/1, Reshape/1
  gets vector from Skew Matrix/1 -> W_retro/1
  Matrix Multiply/1 -> gets vector from Skew Matrix/1
  Derivative/1 -> Matrix Multiply/1
  Transpose/1 -> Derivative/1
  Reshape/1 -> Transpose/1, Matrix Multiply/2

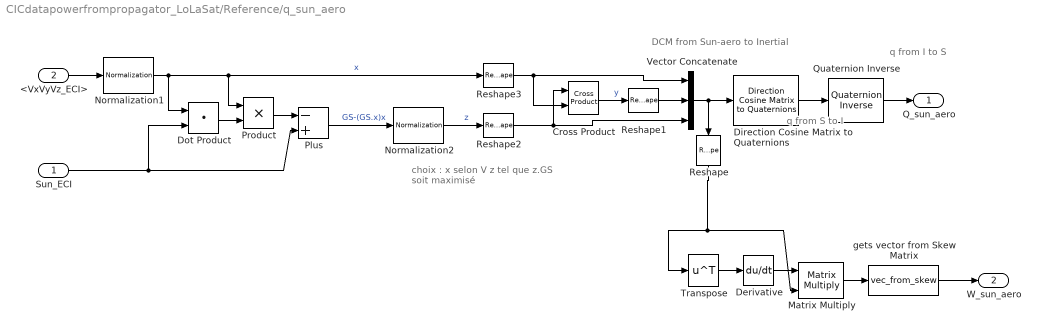
== system CICdatapowerfrompropagator_LoLaSat/Reference/q_sun_aero ==
  note: q from I to S
  note: q from S to I
  note: DCM from Sun-aero to Inertial
  note: choix :
      | x selon V
      | z tel que z.GS soit maximisé
  Sun_ECI : Inport
  <VxVyVz_ECI> : Inport  Port=2
  Cross Product : vrlib/Utilities/Cross Product
  Derivative : Derivative
  Direction Cosine Matrix to Quaternions : sharedtransform/Direction Cosine Matrix  to Quaternions  aMode=0  action=None  tolerance=eps(2)
  Dot Product : DotProduct  OutDataTypeStr=Inherit: Inherit via internal rule
  Matrix Multiply : Product  Multiplication=Matrix(*)
  Normalization1 : dspmathops/Normalization  NormType=2-norm  Bias=1e-10  NormOver=Each column  Dimension=1  roundingMode=Floor  overflowMode=off  accumDataTypeStr=Inherit: Same as product output  accumLastDataTypeStr=Inherit: Same as product output  outputDataTypeStr=Inherit: Same as product output  outputMin=[]  outputMax=[]  outputLastDataTypeStr=Inherit: Same as product output
  Normalization2 : dspmathops/Normalization  NormType=2-norm  Bias=1e-10  NormOver=Each column  Dimension=1  roundingMode=Floor  overflowMode=off  accumDataTypeStr=Inherit: Same as product output  accumLastDataTypeStr=Inherit: Same as product output  outputDataTypeStr=Inherit: Same as product output  outputMin=[]  outputMax=[]  outputLastDataTypeStr=Inherit: Same as product output
  Plus : Sum  Inputs=-+
  Product : Product
  Quaternion Inverse : aerolibutil/Quaternion Inverse
  Reshape : Reshape  OutputDimensionality=Customize  OutputDimensions=[3,3]
  Reshape1 : Reshape  OutputDimensionality=Column vector (2-D)
  Reshape2 : Reshape  OutputDimensionality=Column vector (2-D)
  Reshape3 : Reshape  OutputDimensionality=Column vector (2-D)
  Transpose : Math  Operator=transpose
  Vector Concatenate : Concatenate  NumInputs=3  Mode=Multidimensional array  ConcatenateDimension=2
  gets vector from Skew Matrix : MATLABFcn  MATLABFcn=vec_from_skew
  Q_sun_aero : Outport  VectorParamsAs1DForOutWhenUnconnected=off
  W_sun_aero : Outport  Port=2
  wires:
  Quaternion Inverse/1 -> Q_sun_aero/1
  Reshape2/1 -> Vector Concatenate/3, Cross Product/1
  Reshape3/1 -> Vector Concatenate/1, Cross Product/2
  Product/1 -> Plus/1
  Dot Product/1 -> Product/2
  Cross Product/1 -> Reshape1/1  "y"
  Normalization2/1 -> Reshape2/1  "z"
  Plus/1 -> Normalization2/1  "GS-(GS.x)x"
  Sun_ECI/1 -> Dot Product/2, Plus/2
  Direction Cosine Matrix to Quaternions/1 -> Quaternion Inverse/1
  Normalization1/1 -> Dot Product/1, Product/1, Reshape3/1  "x"
  <VxVyVz_ECI>/1 -> Normalization1/1
  Reshape1/1 -> Vector Concatenate/2
  Transpose/1 -> Derivative/1
  Matrix Multiply/1 -> gets vector from Skew Matrix/1
  Derivative/1 -> Matrix Multiply/1
  Vector Concatenate/1 -> Direction Cosine Matrix to Quaternions/1, Reshape/1
  gets vector from Skew Matrix/1 -> W_sun_aero/1
  Reshape/1 -> Transpose/1, Matrix Multiply/2

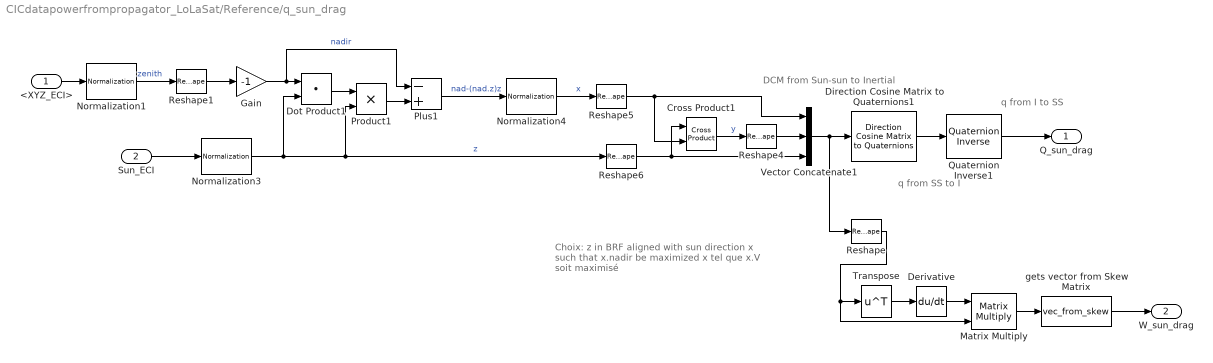
== system CICdatapowerfrompropagator_LoLaSat/Reference/q_sun_drag ==
  note: Choix:
      | z in BRF aligned with sun direction
      | x such that x.nadir be maximized
      | x tel que x.V soit maximisé
  note: DCM from Sun-sun to Inertial
  note: q from I to SS
  note: q from SS to I
  <XYZ_ECI> : Inport
  Sun_ECI : Inport  Port=2
  Cross Product1 : vrlib/Utilities/Cross Product
  Derivative : Derivative
  Direction Cosine Matrix to Quaternions1 : sharedtransform/Direction Cosine Matrix  to Quaternions  aMode=0  action=None  tolerance=eps(2)
  Dot Product1 : DotProduct  OutDataTypeStr=Inherit: Inherit via internal rule
  Gain : Gain  Gain=-1
  Matrix Multiply : Product  Multiplication=Matrix(*)
  Normalization1 : dspmathops/Normalization  NormType=2-norm  Bias=1e-10  NormOver=Each column  Dimension=1  roundingMode=Floor  overflowMode=off  accumDataTypeStr=Inherit: Same as product output  accumLastDataTypeStr=Inherit: Same as product output  outputDataTypeStr=Inherit: Same as product output  outputMin=[]  outputMax=[]  outputLastDataTypeStr=Inherit: Same as product output
  Normalization3 : dspmathops/Normalization  NormType=2-norm  Bias=1e-10  NormOver=Each column  Dimension=1  roundingMode=Floor  overflowMode=off  accumDataTypeStr=Inherit: Same as product output  accumLastDataTypeStr=Inherit: Same as product output  outputDataTypeStr=Inherit: Same as product output  outputMin=[]  outputMax=[]  outputLastDataTypeStr=Inherit: Same as product output
  Normalization4 : dspmathops/Normalization  NormType=2-norm  Bias=1e-10  NormOver=Each column  Dimension=1  roundingMode=Floor  overflowMode=off  accumDataTypeStr=Inherit: Same as product output  accumLastDataTypeStr=Inherit: Same as product output  outputDataTypeStr=Inherit: Same as product output  outputMin=[]  outputMax=[]  outputLastDataTypeStr=Inherit: Same as product output
  Plus1 : Sum  Inputs=-+
  Product1 : Product
  Quaternion Inverse1 : aerolibutil/Quaternion Inverse
  Reshape : Reshape  OutputDimensionality=Customize  OutputDimensions=[3,3]
  Reshape{1,4..6} (4 alike) : Reshape  OutputDimensionality=Column vector (2-D)
  Transpose : Math  Operator=transpose
  Vector Concatenate1 : Concatenate  NumInputs=3  Mode=Multidimensional array  ConcatenateDimension=2
  gets vector from Skew Matrix : MATLABFcn  MATLABFcn=vec_from_skew
  Q_sun_drag : Outport  VectorParamsAs1DForOutWhenUnconnected=off
  W_sun_drag : Outport  Port=2
  wires:
  Direction Cosine Matrix to Quaternions1/1 -> Quaternion Inverse1/1
  Reshape4/1 -> Vector Concatenate1/2
  Dot Product1/1 -> Product1/1
  Sun_ECI/1 -> Normalization3/1
  Quaternion Inverse1/1 -> Q_sun_drag/1
  Reshape1/1 -> Gain/1
  Plus1/1 -> Normalization4/1  "nad-(nad.z)z"
  Reshape6/1 -> Cross Product1/1, Vector Concatenate1/3
  Normalization3/1 -> Dot Product1/2, Product1/2, Reshape6/1  "z"
  Reshape5/1 -> Cross Product1/2, Vector Concatenate1/1
  Cross Product1/1 -> Reshape4/1  "y"
  Normalization4/1 -> Reshape5/1  "x"
  Product1/1 -> Plus1/2
  Reshape/1 -> Matrix Multiply/2, Transpose/1
  Derivative/1 -> Matrix Multiply/1
  Transpose/1 -> Derivative/1
  Matrix Multiply/1 -> gets vector from Skew Matrix/1
  gets vector from Skew Matrix/1 -> W_sun_drag/1
  Vector Concatenate1/1 -> Direction Cosine Matrix to Quaternions1/1, Reshape/1
  <XYZ_ECI>/1 -> Normalization1/1
  Normalization1/1 -> Reshape1/1  "zenith"
  Gain/1 -> Dot Product1/1, Plus1/1  "nadir"

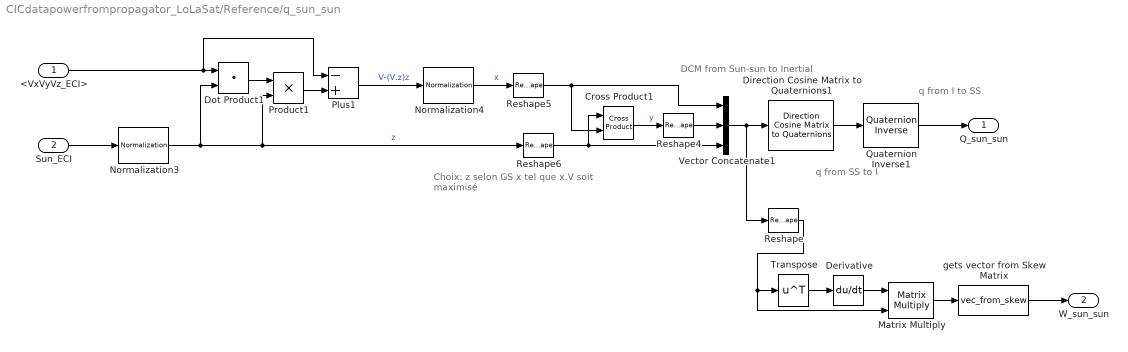
== system CICdatapowerfrompropagator_LoLaSat/Reference/q_sun_sun ==
  note: Choix:
      | z selon GS
      | x tel que x.V soit maximisé
  note: DCM from Sun-sun to Inertial
  note: q from I to SS
  note: q from SS to I
  <VxVyVz_ECI> : Inport
  Sun_ECI : Inport  Port=2
  Cross Product1 : vrlib/Utilities/Cross Product
  Derivative : Derivative
  Direction Cosine Matrix to Quaternions1 : sharedtransform/Direction Cosine Matrix  to Quaternions  aMode=0  action=None  tolerance=eps(2)
  Dot Product1 : DotProduct  OutDataTypeStr=Inherit: Inherit via internal rule
  Matrix Multiply : Product  Multiplication=Matrix(*)
  Normalization3 : dspmathops/Normalization  NormType=2-norm  Bias=1e-10  NormOver=Each column  Dimension=1  roundingMode=Floor  overflowMode=off  accumDataTypeStr=Inherit: Same as product output  accumLastDataTypeStr=Inherit: Same as product output  outputDataTypeStr=Inherit: Same as product output  outputMin=[]  outputMax=[]  outputLastDataTypeStr=Inherit: Same as product output
  Normalization4 : dspmathops/Normalization  NormType=2-norm  Bias=1e-10  NormOver=Each column  Dimension=1  roundingMode=Floor  overflowMode=off  accumDataTypeStr=Inherit: Same as product output  accumLastDataTypeStr=Inherit: Same as product output  outputDataTypeStr=Inherit: Same as product output  outputMin=[]  outputMax=[]  outputLastDataTypeStr=Inherit: Same as product output
  Plus1 : Sum  Inputs=-+
  Product1 : Product
  Quaternion Inverse1 : aerolibutil/Quaternion Inverse
  Reshape : Reshape  OutputDimensionality=Customize  OutputDimensions=[3,3]
  Reshape4 : Reshape  OutputDimensionality=Column vector (2-D)
  Reshape5 : Reshape  OutputDimensionality=Column vector (2-D)
  Reshape6 : Reshape  OutputDimensionality=Column vector (2-D)
  Transpose : Math  Operator=transpose
  Vector Concatenate1 : Concatenate  NumInputs=3  Mode=Multidimensional array  ConcatenateDimension=2
  gets vector from Skew Matrix : MATLABFcn  MATLABFcn=vec_from_skew
  Q_sun_sun : Outport  VectorParamsAs1DForOutWhenUnconnected=off
  W_sun_sun : Outport  Port=2
  wires:
  Direction Cosine Matrix to Quaternions1/1 -> Quaternion Inverse1/1
  Reshape4/1 -> Vector Concatenate1/2
  Dot Product1/1 -> Product1/1
  Sun_ECI/1 -> Normalization3/1
  Quaternion Inverse1/1 -> Q_sun_sun/1
  <VxVyVz_ECI>/1 -> Dot Product1/1, Plus1/1
  Plus1/1 -> Normalization4/1  "V-(V.z)z"
  Reshape6/1 -> Cross Product1/1, Vector Concatenate1/3
  Normalization3/1 -> Dot Product1/2, Product1/2, Reshape6/1  "z"
  Reshape5/1 -> Cross Product1/2, Vector Concatenate1/1
  Cross Product1/1 -> Reshape4/1  "y"
  Normalization4/1 -> Reshape5/1  "x"
  Product1/1 -> Plus1/2
  Reshape/1 -> Matrix Multiply/2, Transpose/1
  Derivative/1 -> Matrix Multiply/1
  Transpose/1 -> Derivative/1
  Matrix Multiply/1 -> gets vector from Skew Matrix/1
  gets vector from Skew Matrix/1 -> W_sun_sun/1
  Vector Concatenate1/1 -> Direction Cosine Matrix to Quaternions1/1, Reshape/1

== matlab function CICdatapowerfrompropagator_LoLaSat/Solar Array & Earth position/MATLAB Function ==
  data: u input; y output
function y = fcn(u)
%Checks if the satellite is in eclipse
% Inputs:
% u(1:3)= position of the satellite in ECI
% u(4:6)= direction of the Sun in ECI
%   
% Output: out=1: S/C in eclipse 
%         out=0: S/C in illumination

%Defining the frames xyz=inertial XYZ=z pointing to sun
Z=u(4:6);
if Z==[0;0;0]
    X=[1;0;0];
else 
    X=[-Z(2);Z(1);0];
end

X=X/norm(X);
Y=cross(Z,X);

R_i2s=[ X'*[1;0;0] , Y'*[1;0;0] , Z'*[1;0;0] ;...
        X'*[0;1;0] , Y'*[0;1;0] , Z'*[0;1;0] ;...
        X'*[0;0;1] , Y'*[0;0;1] , Z'*[0;0;1] ];
%position of the satellite in new frame XYZ=z pointing to sun    
r_s=R_i2s'*u(1:3);
a=r_s(1);
b=r_s(2);
c=r_s(3);
%check if satellite is in shadow: shadow=0
if c<0
    if ((b^2)+(a^2))<4.0678884e+13
        y=1.0;
    else
        y=0.0;
    end
else
    y=0.0;
end

== matlab function CICdatapowerfrompropagator_LoLaSat/get LLA/ECI To LLA ==
  data: X_ECEF input; h output; lat output; long output
function [h, lat, long] = fcn(X_ECEF)
    h = 0;
    lat = 0;
    long = 0;
[lat, long, h] = ecef2geod(X_ECEF(1),X_ECEF(2),X_ECEF(3));

== matlab function CICdatapowerfrompropagator_LoLaSat/get LLA/JD to UTC ==
  data: JD input; Time_UTC output
function Time_UTC = fcn(JD)
    coder.extrinsic('datetime','datevec');
    Time_UTC = [0,0,0,0,0,0];
Time_UTC =  datevec(datetime(JD,'convertfrom','juliandate'));
